simulink model "test_current"  (R2024b)
settings: Solver=ode4  StartTime=0.0  StopTime=0.05  FixedStep=1e-5  RelTol=1e-3
values from neighbouring files (symbols this model uses):
  B = 0.001    [step5a_plant.m]    (also in step5b_current_control.m; step5c_speed_control.m; step5d_position_control.m)
  J = 0.01    [step5a_plant.m]    (also in step5b_current_control.m; step5c_speed_control.m; step5d_position_control.m)
  Ki_id = 800.0    (= 800)    [simulate_surface_pmsm_foc.m]    (also in step2_build_current_loop_svpwm.m = 2 * pi * f_bw_id * Rs; step3_build_speed_loop.m = 2 * pi * f_bw_id * Rs; step4_build_position_loop.m = 2 * pi * 500 * Rs; step5b_current_control.m = 9424.77796077)
  Ki_iq = 800.0    (= 800)    [simulate_surface_pmsm_foc.m]    (also in step2_build_current_loop_svpwm.m = 2 * pi * f_bw_iq * Rs; step3_build_speed_loop.m = 2 * pi * f_bw_iq * Rs; step4_build_position_loop.m = 2 * pi * 500 * Rs; step5b_current_control.m = 9424.77796077)
  Kp_id = 40.0    (= 40)    [simulate_surface_pmsm_foc.m]    (also in step2_build_current_loop_svpwm.m = 2 * pi * f_bw_id * Ld_nom; step3_build_speed_loop.m = 2 * pi * f_bw_id * Ld_nom; step4_build_position_loop.m = 2 * pi * 500 * Ld_nom; step5b_current_control.m = 3.14159265359)
  Kp_iq = 40.0    (= 40)    [simulate_surface_pmsm_foc.m]    (also in step2_build_current_loop_svpwm.m = 2 * pi * f_bw_iq * Lq_nom; step3_build_speed_loop.m = 2 * pi * f_bw_iq * Lq_nom; step4_build_position_loop.m = 2 * pi * 500 * Lq_nom; step5b_current_control.m = 3.14159265359)
  Ld_nom = 0.001    [step5a_plant.m]    (also in step5b_current_control.m; step5c_speed_control.m; step5d_position_control.m)
  Lq_nom = 0.001    [step5a_plant.m]    (also in step5b_current_control.m; step5c_speed_control.m; step5d_position_control.m)
  PolePairs = 3    [step5a_plant.m]    (also in step5b_current_control.m; step5c_speed_control.m; step5d_position_control.m)
  psi_d_nom = 0.08    [step5a_plant.m]    (also in step5b_current_control.m; step5c_speed_control.m; step5d_position_control.m)
  Rs = interp1(obj.TempGrid, obj.RsMap, temperature, 'linear', 'extrap')    [SurfaceMountedPMSM.m]    (also in simulate_surface_pmsm_foc.m = motor.interpRs(temperature); step1_build_plant_openloop.m = motor.interpRs(temperature); step2_build_current_loop_svpwm.m = motor.interpRs(temperature); step3_build_speed_loop.m = motor.interpRs(temperature))
settings Model: Creator=Lee  LastModifiedBy=Lee

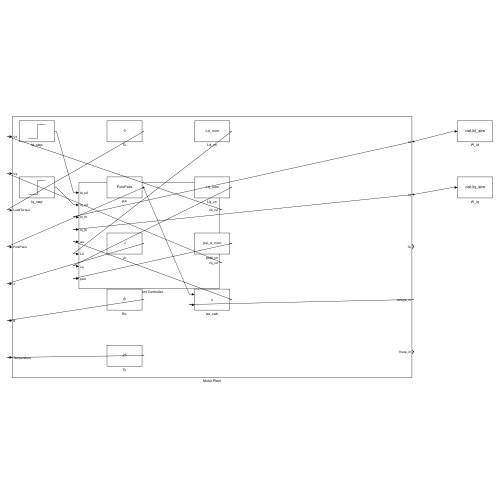
[thumbnail: Simulink's stored preview of the top-level diagram]
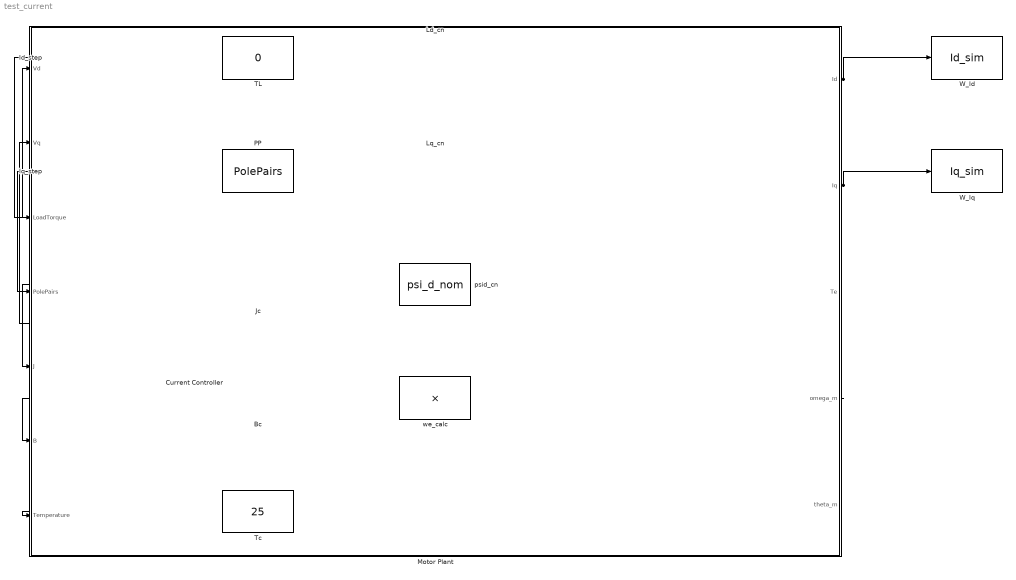
== system test_current ==
  Bc : Constant  Value=B
  Current Controller : Subsystem
  Id_step : Step  Time=0  SampleTime=0
  Iq_step : Step  Time=0.01  After=2  SampleTime=0
  Jc : Constant  Value=J
  Ld_cn : Constant  Value=Ld_nom
  Lq_cn : Constant  Value=Lq_nom
  Motor Plant : Subsystem
  PP : Constant  Value=PolePairs
  TL : Constant  Value=0
  Tc : Constant  Value=25
  W_Id : ToWorkspace  VariableName=Id_sim  SampleTime=-1
  W_Iq : ToWorkspace  VariableName=Iq_sim  SampleTime=-1
  psid_cn : Constant  Value=psi_d_nom
  we_calc : Product
  wires:
  Id_step/1 -> Current Controller/1(Id_ref)
  Iq_step/1 -> Current Controller/2(Iq_ref)
  Motor Plant/1(Id) -> Current Controller/3(Id_fb), W_Id/1
  Motor Plant/2(Iq) -> Current Controller/4(Iq_fb), W_Iq/1
  we_calc/1 -> Current Controller/5(we)
  Ld_cn/1 -> Current Controller/6(Ld)
  Lq_cn/1 -> Current Controller/7(Lq)
  psid_cn/1 -> Current Controller/8(psid)
  Current Controller/1(Vd_ref) -> Motor Plant/1(Vd)
  Current Controller/2(Vq_ref) -> Motor Plant/2(Vq)
  PP/1 -> we_calc/1, Motor Plant/4(PolePairs)
  Motor Plant/4(omega_m) -> we_calc/2
  TL/1 -> Motor Plant/3(LoadTorque)
  Jc/1 -> Motor Plant/5(J)
  Bc/1 -> Motor Plant/6(B)
  Tc/1 -> Motor Plant/7(Temperature)

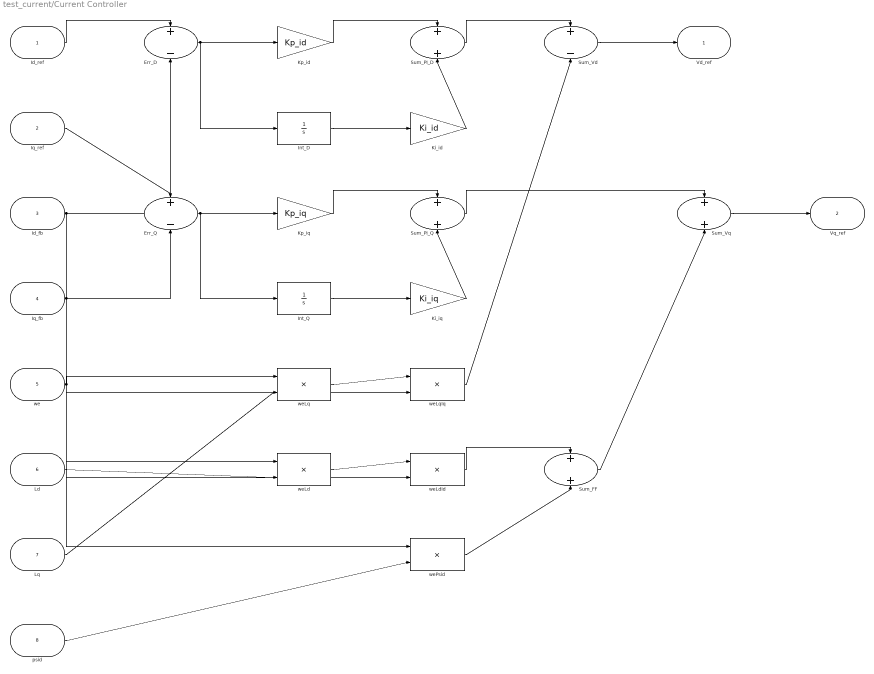
== system test_current/Current Controller ==
  Id_ref : Inport
  Iq_ref : Inport  Port=2
  Id_fb : Inport  Port=3
  Iq_fb : Inport  Port=4
  we : Inport  Port=5
  Ld : Inport  Port=6
  Lq : Inport  Port=7
  psid : Inport  Port=8
  Err_D : Sum  Inputs=+-
  Err_Q : Sum  Inputs=+-
  Int_D : Integrator
  Int_Q : Integrator
  Ki_id : Gain  Gain=Ki_id
  Ki_iq : Gain  Gain=Ki_iq
  Kp_id : Gain  Gain=Kp_id
  Kp_iq : Gain  Gain=Kp_iq
  Sum_FF : Sum
  Sum_PI_D : Sum
  Sum_PI_Q : Sum
  Sum_Vd : Sum  Inputs=+-
  Sum_Vq : Sum
  weLd : Product
  weLdId : Product
  weLq : Product
  weLqIq : Product
  wePsid : Product
  Vd_ref : Outport
  Vq_ref : Outport  Port=2
  wires:
  ? -> ?
  Id_ref/1 -> Err_D/1
  Id_fb/1 -> Err_D/2, weLdId/2
  Err_D/1 -> Kp_id/1, Int_D/1
  Int_D/1 -> Ki_id/1
  Kp_id/1 -> Sum_PI_D/1
  Ki_id/1 -> Sum_PI_D/2
  we/1 -> weLq/1, weLd/1, wePsid/1
  Lq/1 -> weLq/2
  weLq/1 -> weLqIq/1
  Iq_fb/1 -> weLqIq/2, Err_Q/2
  Sum_PI_D/1 -> Sum_Vd/1
  weLqIq/1 -> Sum_Vd/2
  Sum_Vd/1 -> Vd_ref/1
  Iq_ref/1 -> Err_Q/1
  Err_Q/1 -> Kp_iq/1, Int_Q/1
  Int_Q/1 -> Ki_iq/1
  Kp_iq/1 -> Sum_PI_Q/1
  Ki_iq/1 -> Sum_PI_Q/2
  Ld/1 -> weLd/2
  weLd/1 -> weLdId/1
  psid/1 -> wePsid/2
  weLdId/1 -> Sum_FF/1
  wePsid/1 -> Sum_FF/2
  Sum_PI_Q/1 -> Sum_Vq/1
  Sum_FF/1 -> Sum_Vq/2
  Sum_Vq/1 -> Vq_ref/1

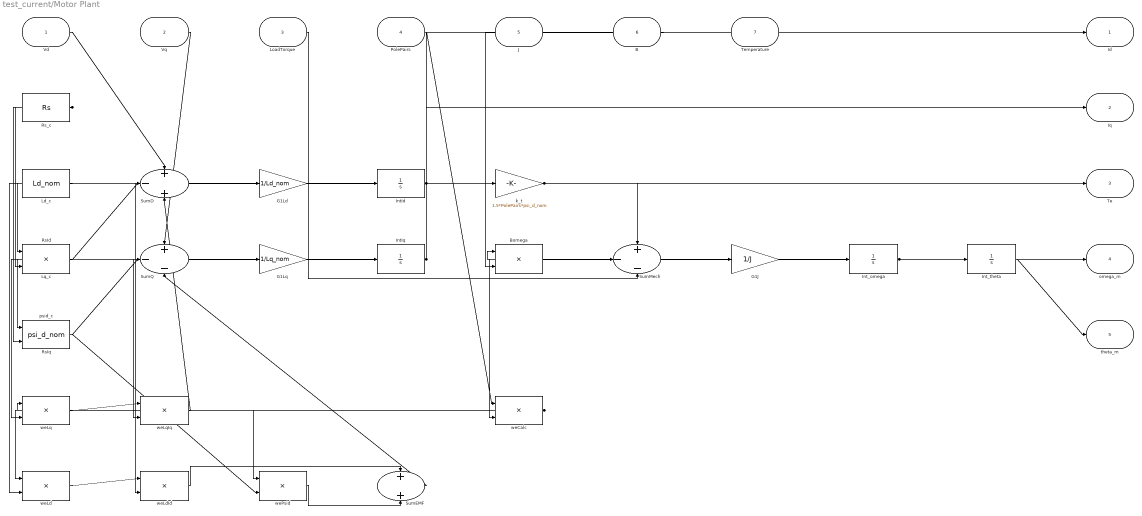
== system test_current/Motor Plant ==
  Vd : Inport
  Vq : Inport  Port=2
  LoadTorque : Inport  Port=3
  PolePairs : Inport  Port=4
  J : Inport  Port=5
  B : Inport  Port=6
  Temperature : Inport  Port=7
  Bomega : Product
  G1J : Gain  Gain=1/J
  G1Ld : Gain  Gain=1/Ld_nom
  G1Lq : Gain  Gain=1/Lq_nom
  IntId : Integrator
  IntIq : Integrator
  Int_omega : Integrator
  Int_theta : Integrator
  Ld_c : Constant  Value=Ld_nom
  Lq_c : Constant  Value=Lq_nom
  RsId : Product
  RsIq : Product
  Rs_c : Constant  Value=Rs
  SumD : Sum  Inputs=+-+
  SumEMF : Sum
  SumMech : Sum  Inputs=+--
  SumQ : Sum  Inputs=+--
  k_t : Gain  Gain=1.5*PolePairs*psi_d_nom
  psid_c : Constant  Value=psi_d_nom
  weCalc : Product
  weLd : Product
  weLdId : Product
  weLq : Product
  weLqIq : Product
  wePsid : Product
  Id : Outport
  Iq : Outport  Port=2
  Te : Outport  Port=3
  omega_m : Outport  Port=4
  theta_m : Outport  Port=5
  wires:
  ? -> ?
  Vd/1 -> SumD/1
  IntId/1 -> RsId/1, Id/1, weLdId/2
  Rs_c/1 -> RsId/2, RsIq/2
  RsId/1 -> SumD/2
  weLqIq/1 -> SumD/3
  SumD/1 -> G1Ld/1
  G1Ld/1 -> IntId/1
  Vq/1 -> SumQ/1
  IntIq/1 -> RsIq/1, Iq/1, weLqIq/2, k_t/1
  RsIq/1 -> SumQ/2
  SumEMF/1 -> SumQ/3
  SumQ/1 -> G1Lq/1
  G1Lq/1 -> IntIq/1
  PolePairs/1 -> weCalc/1
  Int_omega/1 -> weCalc/2, Bomega/1, Int_theta/1, omega_m/1
  weCalc/1 -> weLq/1, weLd/1, wePsid/1
  Lq_c/1 -> weLq/2
  weLq/1 -> weLqIq/1
  Ld_c/1 -> weLd/2
  weLd/1 -> weLdId/1
  psid_c/1 -> wePsid/2
  weLdId/1 -> SumEMF/1
  wePsid/1 -> SumEMF/2
  k_t/1 -> SumMech/1, Te/1
  B/1 -> Bomega/2
  Bomega/1 -> SumMech/2
  LoadTorque/1 -> SumMech/3
  SumMech/1 -> G1J/1
  G1J/1 -> Int_omega/1
  Int_theta/1 -> theta_m/1
